simulink model "robot_serie"  (R2020a)
settings: Solver=VariableStepAuto  StartTime=0.0  StopTime=2  FixedStep=0.001  MaxStep=10^-3  MinStep=10^-4  RelTol=1e-3
values from neighbouring files (symbols this model uses):
  q0 = homeConfiguration(robot)    [sim_robSerie.m]
  robot = importrobot('..\Simulacion dinamica brazo\Modelos urdf brazo\Robot\urdf\Robot.urdf')    [sim_robSerie.m]
  weights = [0, 0, 0, 1, 1, 1]    [sim_robSerie.m]
libraries: robotmaniplib x6, simulink x2
settings Model: Creator=Rodrigo  LastModifiedBy=Rodrigo

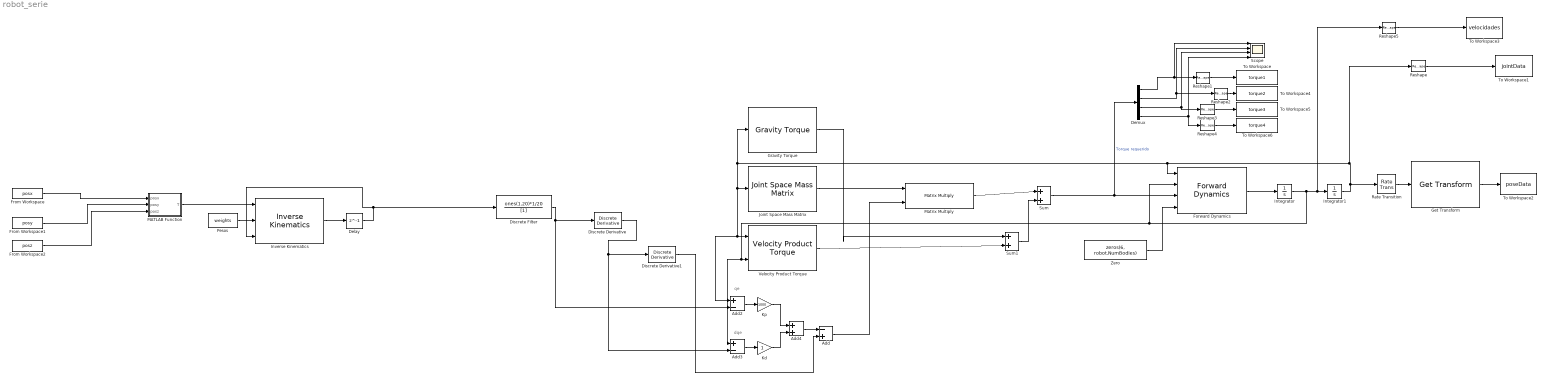
== system robot_serie ==
  note: dqe
  note: qe
  Add : Sum  Inputs=-+
  Add2 : Sum  Inputs=+-
  Add3 : Sum  Inputs=+-
  Add4 : Sum
  Delay : Delay  DelayLength=1
  Demux : Demux
  Discrete Derivative : simulink/Discrete/Discrete Derivative  gainval=1.0  ICPrevScaledInput=0.0  OutMin=[]  OutMax=[]  OutDataType=fixdt(1, 16)  OutScaling=2^-10  DoSatur=off
  Discrete Derivative1 : simulink/Discrete/Discrete Derivative  gainval=1.0  ICPrevScaledInput=0.0  OutMin=[]  OutMax=[]  OutDataType=fixdt(1, 16)  OutScaling=2^-10  DoSatur=off
  Discrete Filter : DiscreteFilter  Numerator=ones(1,20)*1/20  Denominator=[1]  InitialStates=repmat(q0',19,1)
  Forward Dynamics : robotmaniplib/Forward Dynamics  RigidBodyTree=robot  SimulateUsing=Interpreted execution
  From Workspace : FromWorkspace  VariableName=posx
  From Workspace1 : FromWorkspace  VariableName=posy
  From Workspace2 : FromWorkspace  VariableName=posz
  Get Transform : robotmaniplib/Get Transform  RigidBodyTree=robot  SourceBody=tool  TargetBody=base_link  SimulateUsing=Interpreted execution
  Gravity Torque : robotmaniplib/Gravity Torque  RigidBodyTree=robot  SimulateUsing=Interpreted execution
  Integrator : Integrator
  Integrator1 : Integrator
  Inverse Kinematics : robotmaniplib/Inverse Kinematics  RigidBodyTree=robot  EndEffector=tool  ShowInfo=off  SolverName=BFGS Gradient Projection  EnforceJointLimits=on  MaxIterations=1500  MaxTime=10  GradientTolerance=1e-7  SolutionTolerance=1e-6  StepTolerance=1e-14  ErrorChangeTolerance=1e-12  UseErrorDamping=on  DampingBias=0.0025  SimulateUsing=Interpreted execution
  Joint Space Mass Matrix : robotmaniplib/Joint Space Mass Matrix  RigidBodyTree=robot  SimulateUsing=Interpreted execution
  Kd : Gain
  Kp : Gain  Gain=1000
  MATLAB Function : MATLAB Function  TreatAsAtomicUnit=on
  Matrix Multiply : Product  Multiplication=Matrix(*)
  Pesos : Constant  Value=weights
  Rate Transition : RateTransition
  Reshape{,1..5} (6 alike) : Reshape
  Scope : Scope  NumInputPorts=4
  Sum : Sum  Inputs=|++
  Sum1 : Sum  Inputs=|++
  To Workspace : ToWorkspace  VariableName=torque1  SaveFormat=Timeseries  SampleTime=-1
  To Workspace1 : ToWorkspace  VariableName=jointData  SampleTime=-1
      settings: Save2DSignal=2-D array (concatenate along first dimension)
  To Workspace2 : ToWorkspace  VariableName=poseData  SampleTime=-1
  To Workspace3 : ToWorkspace  VariableName=velocidades  SampleTime=-1
      settings: Save2DSignal=2-D array (concatenate along first dimension)
  To Workspace4 : ToWorkspace  VariableName=torque2  SaveFormat=Timeseries  SampleTime=-1
  To Workspace5 : ToWorkspace  VariableName=torque3  SaveFormat=Timeseries  SampleTime=-1
  To Workspace6 : ToWorkspace  VariableName=torque4  SaveFormat=Timeseries  SampleTime=-1
  Velocity Product Torque : robotmaniplib/Velocity Product Torque  RigidBodyTree=robot  SimulateUsing=Interpreted execution
      settings: SourceProductBaseCode=RO
  Zero : Constant  Value=zeros(6, robot.NumBodies)  OutDataTypeStr=Inherit: Inherit via back propagation
  wires:
  Pesos/1 -> Inverse Kinematics/2
  Rate Transition/1 -> Get Transform/1
  Inverse Kinematics/1 -> Delay/1
  Joint Space Mass Matrix/1 -> Matrix Multiply/1
  Discrete Derivative1/1 -> Add/2
  Add3/1 -> Kd/1
  Integrator/1 -> Forward Dynamics/2, Add3/1, Velocity Product Torque/2, Reshape5/1, Integrator1/1
  Kp/1 -> Add4/1
  Discrete Derivative/1 -> Discrete Derivative1/1, Add3/2
  Add4/1 -> Add/1
  Add2/1 -> Kp/1
  Kd/1 -> Add4/2
  Discrete Filter/1 -> Discrete Derivative/1, Add2/2
  Add/1 -> Matrix Multiply/2
  Forward Dynamics/1 -> Integrator/1
  Matrix Multiply/1 -> Sum/1
  Velocity Product Torque/1 -> Sum1/2
  Gravity Torque/1 -> Sum1/1
  Sum1/1 -> Sum/2
  Sum/1 -> Forward Dynamics/3, Demux/1  "Torque requerido"
  Zero/1 -> Forward Dynamics/4
  Get Transform/1 -> To Workspace2/1
  Reshape/1 -> To Workspace1/1
  Integrator1/1 -> Reshape/1, Forward Dynamics/1, Gravity Torque/1, Velocity Product Torque/1, Add2/1, Joint Space Mass Matrix/1, Rate Transition/1
  MATLAB Function/1(T) -> Inverse Kinematics/1
  Demux/1 -> Scope/1, Reshape1/1
  Demux/2 -> Scope/2, Reshape2/1
  Demux/3 -> Reshape3/1, Scope/3
  Demux/4 -> Reshape4/1, Scope/4
  From Workspace/1 -> MATLAB Function/1(posx)
  From Workspace1/1 -> MATLAB Function/2(posy)
  From Workspace2/1 -> MATLAB Function/3(posz)
  Delay/1 -> Inverse Kinematics/3, Discrete Filter/1
  Reshape1/1 -> To Workspace/1
  Reshape2/1 -> To Workspace4/1
  Reshape3/1 -> To Workspace5/1
  Reshape4/1 -> To Workspace6/1
  Reshape5/1 -> To Workspace3/1

== matlab function robot_serie/MATLAB Function ==
  data: posx input; T output; posy input; posz input
function T = fcn(posx,posy,posz)
pos = [posx,posy,posz];
T=trvec2tform(pos);
